simulink model "acc"  (R2025a)
settings: Solver=VariableStepAuto  StartTime=0.0  StopTime=10.0  RelTol=1e-3
settings Model: Creator=sanborkl  LastModifiedBy=sanborkl

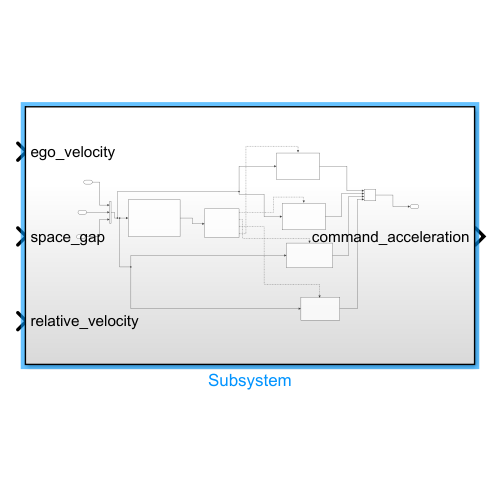
[thumbnail: Simulink's stored preview of the top-level diagram]
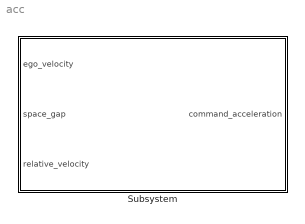
== system acc ==
  Subsystem : Subsystem

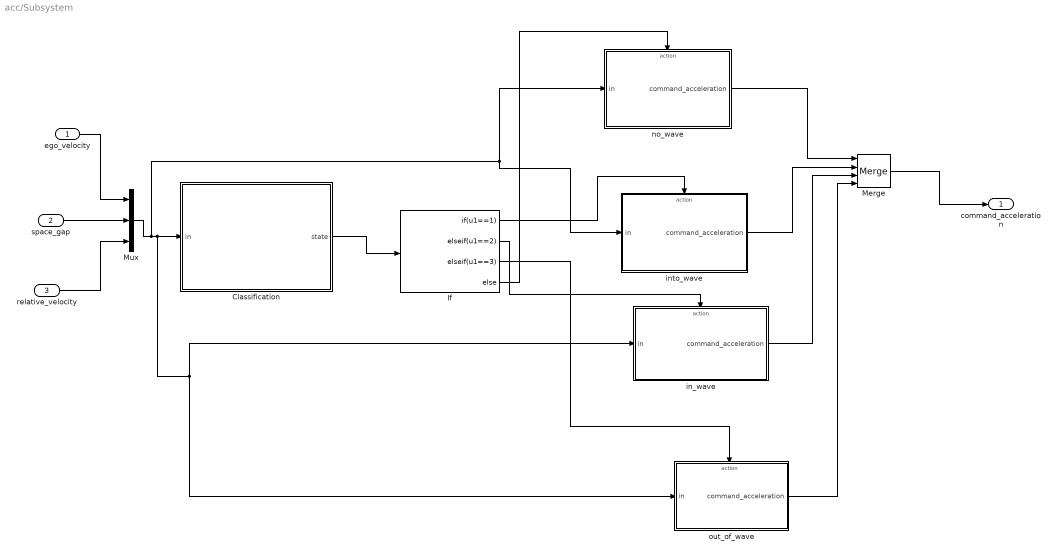
== system acc/Subsystem ==
  ego_velocity : Inport
  space_gap : Inport  Port=2
  relative_velocity : Inport  Port=3
  Classification : Subsystem
  If : If  IfExpression=u1==1  ElseIfExpressions=u1==2,u1==3
  Merge : Merge  Inputs=4
  Mux : Mux  Inputs=3
  in_wave : Subsystem  TreatAsAtomicUnit=on
  into_wave : Subsystem  TreatAsAtomicUnit=on
  no_wave : Subsystem  TreatAsAtomicUnit=on
  out_of_wave : Subsystem  TreatAsAtomicUnit=on
  command_acceleration : Outport
  wires:
  Classification/1(state) -> If/1
  ego_velocity/1 -> Mux/1
  space_gap/1 -> Mux/2
  relative_velocity/1 -> Mux/3
  Mux/1 -> into_wave/1(in), no_wave/1(in), out_of_wave/1(in), in_wave/1(in), Classification/1(in)
  no_wave/1(command_acceleration) -> Merge/1
  into_wave/1(command_acceleration) -> Merge/2
  in_wave/1(command_acceleration) -> Merge/3
  Merge/1 -> command_acceleration/1
  If/1 -> into_wave/Action
  If/2 -> in_wave/Action
  If/3 -> out_of_wave/Action
  If/4 -> no_wave/Action
  out_of_wave/1(command_acceleration) -> Merge/4

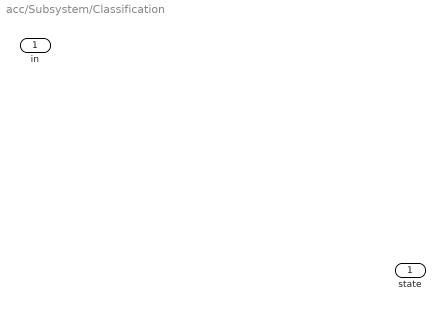
== system acc/Subsystem/Classification ==
  in : Inport
  state : Outport

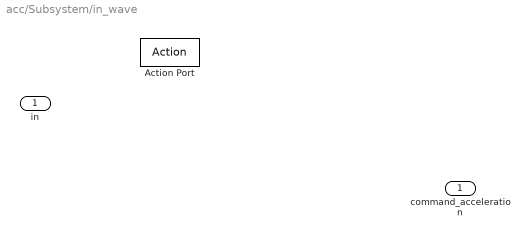
== system acc/Subsystem/in_wave ==
  in : Inport
  Action Port : ActionPort  ActionPortLabel=elseif(u1==2)
  command_acceleration : Outport

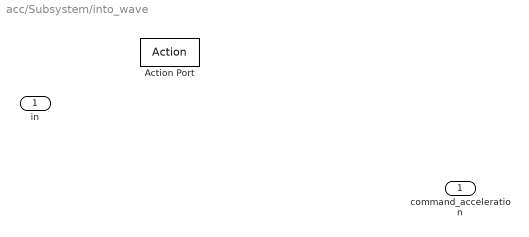
== system acc/Subsystem/into_wave ==
  in : Inport
  Action Port : ActionPort  ActionPortLabel=if(u1==1)
  command_acceleration : Outport

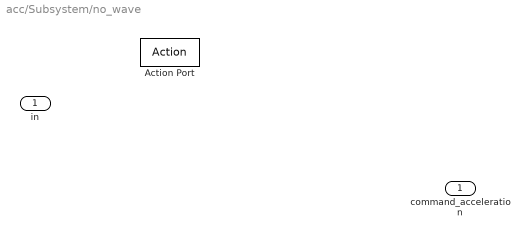
== system acc/Subsystem/no_wave ==
  in : Inport
  Action Port : ActionPort  ActionPortLabel=else
  command_acceleration : Outport

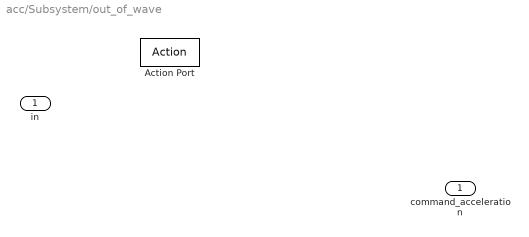
== system acc/Subsystem/out_of_wave ==
  in : Inport
  Action Port : ActionPort  ActionPortLabel=elseif(u1==3)
  command_acceleration : Outport
